simulink model "sampleModel1769"  (R2023a)
settings: Solver=VariableStepAuto  StartTime=0.0  StopTime=10.0  RelTol=1e-3
libraries: hdlsllib x5, simulink x1
settings Model: Creator=user1  LastModifiedBy=user1

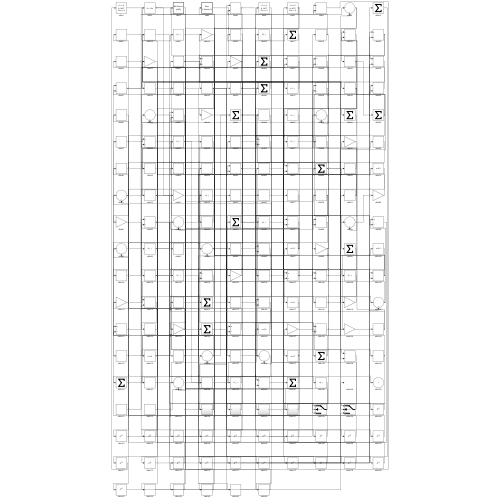
[thumbnail: Simulink's stored preview of the top-level diagram]
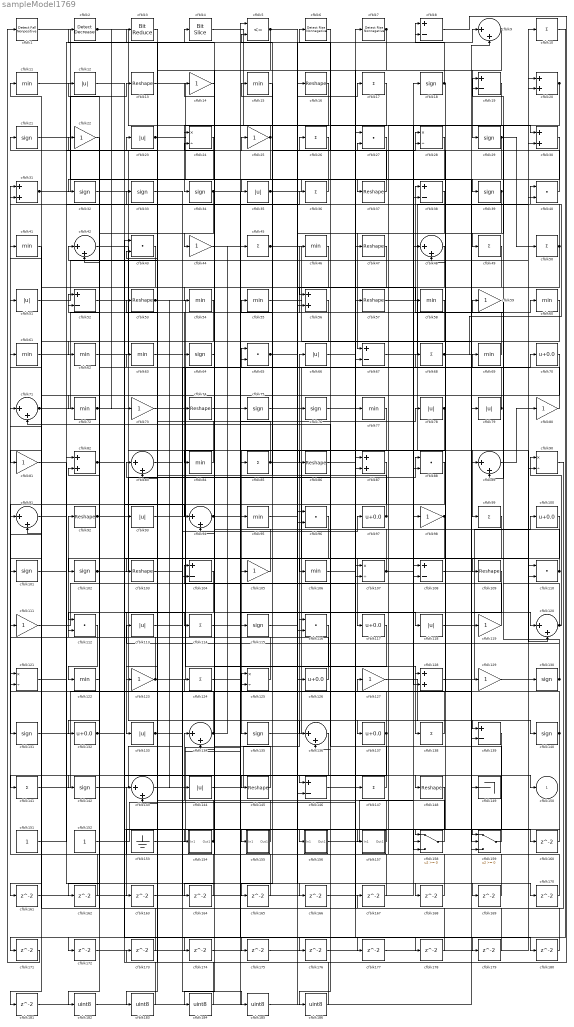
== system sampleModel1769 ==
  cfblk1 : hdlsllib/Logic and Bit Operations/Detect Fall Nonpositive  vinit=0  OutDataTypeStr=boolean
  cfblk{10,17,26,36,45,49..50,68,85,99,114,124,138,141,147} (15 alike) : Sum  Inputs=+
  cfblk{70,97,100,117,126,132,137} (7 alike) : Bias  Bias=0.0  SaturateOnIntegerOverflow=off
  cfblk{18,21,29,32..34,39,64,75..76,101..102,115,130..131,135,140,142} (18 alike) : Signum
  cfblk{13,16,37,47,53,57,74,86,92,103,109,145,148} (13 alike) : Reshape
  cfblk{8,19,38,52,67,104,108,139,146} (9 alike) : Sum  Inputs=+-
  cfblk{14,22,25,44,59,73,80..81,98,105,111,119,123,127,129} (15 alike) : Gain
  cfblk{11,15,41,46,54..55,58,60..63,69,72,77,84,95,106,122} (18 alike) : MinMax
  cfblk{24,28,90,107,121,125} (6 alike) : Product  Inputs=*/  RndMeth=Zero  SaturateOnIntegerOverflow=on
  cfblk{27,40,43,65,88,96,110,112,116} (9 alike) : DotProduct  OutDataTypeStr=Inherit: Inherit via internal rule
  cfblk{12,23,35,51,66,78..79,93,113,118,133,144} (12 alike) : Abs  SaturateOnIntegerOverflow=off
  cfblk{9,42,48,71,83,89,91,94,120,134,136,143} (12 alike) : Sum  Inputs=|++
  cfblk{20,30..31,56,82,87,128} (7 alike) : Sum
  cfblk149 : Terminator
  cfblk151 : Constant  SampleTime=-1
  cfblk152 : Constant  SampleTime=-1
  cfblk153 : Ground
  cfblk154 : Subsystem
      settings: LibrarySourceBlock=|
      | hdlsllib/Ports &
      | Subsystems/Subsystem
  cfblk155 : Subsystem
      settings: LibrarySourceBlock=|
      | hdlsllib/Ports &
      | Subsystems/Subsystem
  cfblk156 : Subsystem
      settings: LibrarySourceBlock=|
      | hdlsllib/Ports &
      | Subsystems/Subsystem
  cfblk157 : Subsystem
      settings: LibrarySourceBlock=|
      | hdlsllib/Ports &
      | Subsystems/Subsystem
  cfblk158 : Switch  SaturateOnIntegerOverflow=off  InputSameDT=off
  cfblk159 : Switch  SaturateOnIntegerOverflow=off  InputSameDT=off
  cfblk{160..181} (22 alike) : Delay  SampleTime=1
  cfblk{182..186} (5 alike) : DataTypeConversion  OutDataTypeStr=uint8  SaturateOnIntegerOverflow=off  RndMeth=Floor
  cfblk2 : simulink/Logic and Bit Operations/Detect Decrease  vinit=0.0  OutDataTypeStr=boolean
      settings: LibrarySourceBlock=|
      | hdlsllib/Logic and Bit
      | Operations/Detect
      | Decrease
  cfblk3 : hdlsllib/Logic and Bit Operations/Bit Reduce  mode=AND
  cfblk4 : hdlsllib/Logic and Bit Operations/Bit Slice  lidx=7  ridx=0
  cfblk5 : RelationalOperator  Operator=<=  OutDataTypeStr=boolean  InputSameDT=off
  cfblk6 : hdlsllib/Logic and Bit Operations/Detect Rise Nonnegative  vinit=0  OutDataTypeStr=boolean
  cfblk7 : hdlsllib/Logic and Bit Operations/Detect Rise Nonnegative  vinit=0  OutDataTypeStr=boolean
  cfblk150 : Outport  VectorParamsAs1DForOutWhenUnconnected=off
  wires:
  cfblk123/1 -> cfblk69/1, cfblk61/1
  cfblk128/1 -> cfblk100/1
  cfblk93/1 -> cfblk60/1
  cfblk77/1 -> cfblk135/1
  cfblk68/1 -> cfblk40/1, cfblk110/2
  cfblk69/1 -> cfblk38/1
  cfblk2/1 -> cfblk30/1, cfblk73/1
  cfblk16/1 -> cfblk34/1
  cfblk157/1(Out1) -> cfblk134/1
  cfblk140/1 -> cfblk68/1, cfblk163/1
  cfblk89/1 -> cfblk80/1
  cfblk85/1 -> cfblk109/1, cfblk8/1, cfblk64/1
  cfblk112/1 -> cfblk122/1
  cfblk97/1 -> cfblk42/1, cfblk21/1, cfblk55/1
  cfblk144/1 -> cfblk66/1
  cfblk31/1 -> cfblk13/1, cfblk28/2
  cfblk26/1 -> cfblk35/1
  cfblk51/1 -> cfblk30/2
  cfblk148/1 -> cfblk31/1
  cfblk133/1 -> cfblk70/1, cfblk83/2
  cfblk38/1 -> cfblk67/1
  cfblk56/1 -> cfblk155/1(In1)
  cfblk88/1 -> cfblk131/1
  cfblk36/1 -> cfblk32/1
  cfblk131/1 -> cfblk79/1
  cfblk34/1 -> cfblk150/1, cfblk72/1, cfblk156/1(In1), cfblk128/1
  cfblk1/1 -> cfblk119/1
  cfblk75/1 -> cfblk16/1
  cfblk32/1 -> cfblk25/1
  cfblk29/1 -> cfblk115/1, cfblk50/1
  cfblk52/1 -> cfblk140/1
  cfblk135/1 -> cfblk10/1
  cfblk145/1 -> cfblk124/1
  cfblk125/1 -> cfblk92/1
  cfblk33/1 -> cfblk136/1
  cfblk136/1 -> cfblk141/1
  cfblk120/1 -> cfblk90/1, cfblk19/1
  cfblk53/1 -> cfblk106/1, cfblk144/1
  cfblk42/1 -> cfblk137/1
  cfblk98/1 -> cfblk117/1, cfblk28/1
  cfblk104/1 -> cfblk133/1
  cfblk23/1 -> cfblk147/1, cfblk77/1
  cfblk127/1 -> cfblk139/1
  cfblk62/1 -> cfblk26/1
  cfblk137/1 -> cfblk127/1, cfblk165/1
  cfblk147/1 -> cfblk83/1
  cfblk11/1 -> cfblk129/1
  cfblk21/1 -> cfblk37/1
  cfblk4/1 -> cfblk98/1
  cfblk45/1 -> cfblk139/2, cfblk58/1
  cfblk102/1 -> cfblk88/1, cfblk175/1
  cfblk153/1 -> cfblk75/1
  cfblk30/1 -> cfblk95/1
  cfblk152/1 -> cfblk7/1
  cfblk142/1 -> cfblk97/1
  cfblk138/1 -> cfblk51/1
  cfblk92/1 -> cfblk93/1, cfblk94/1
  cfblk114/1 -> cfblk118/1
  cfblk155/1(Out1) -> cfblk53/1
  cfblk100/1 -> cfblk102/1
  cfblk5/1 -> cfblk94/2, cfblk168/1
  cfblk65/1 -> cfblk90/2, cfblk5/2
  cfblk154/1(Out1) -> cfblk121/1, cfblk111/1
  cfblk15/1 -> cfblk145/1
  cfblk67/1 -> cfblk20/2
  cfblk79/1 -> cfblk23/1, cfblk22/1
  cfblk141/1 -> cfblk116/1
  cfblk80/1 -> cfblk12/1
  cfblk109/1 -> cfblk142/1
  cfblk132/1 -> cfblk125/1, cfblk158/2
  cfblk129/1 -> cfblk130/1
  cfblk95/1 -> cfblk17/1
  cfblk25/1 -> cfblk54/1, cfblk112/1, cfblk24/1
  cfblk57/1 -> cfblk99/1
  cfblk151/1 -> cfblk82/1
  cfblk27/1 -> cfblk123/1
  cfblk73/1 -> cfblk138/1
  cfblk84/1 -> cfblk33/1
  cfblk72/1 -> cfblk132/1, cfblk120/2, cfblk148/1
  cfblk110/1 -> cfblk74/1, cfblk14/1
  cfblk9/1 -> cfblk84/1, cfblk29/1
  cfblk156/1(Out1) -> cfblk48/1
  cfblk78/1 -> cfblk96/2, cfblk128/2
  cfblk83/1 -> cfblk65/1
  cfblk3/1 -> cfblk103/1
  cfblk12/1 -> cfblk146/1
  cfblk116/1 -> cfblk146/2
  cfblk134/1 -> cfblk82/2, cfblk45/1
  cfblk35/1 -> cfblk39/1, cfblk158/3
  cfblk17/1 -> cfblk136/2
  cfblk76/1 -> cfblk47/1
  cfblk115/1 -> cfblk76/1
  cfblk7/1 -> cfblk87/2, cfblk183/1
  cfblk119/1 -> cfblk104/1
  cfblk159/1 -> cfblk71/2
  cfblk50/1 -> cfblk154/1(In1), cfblk11/1, cfblk19/2
  cfblk96/1 -> cfblk143/2
  cfblk20/1 -> cfblk157/1(In1), cfblk49/1
  cfblk86/1 -> cfblk107/1
  cfblk41/1 -> cfblk81/1
  cfblk28/1 -> cfblk105/1
  cfblk122/1 -> cfblk52/1
  cfblk111/1 -> cfblk57/1
  cfblk130/1 -> cfblk59/1, cfblk113/1
  cfblk61/1 -> cfblk38/2
  cfblk94/1 -> cfblk169/1, cfblk170/1
  cfblk143/1 -> cfblk85/1
  cfblk71/1 -> cfblk46/1, cfblk31/2
  cfblk158/1 -> cfblk4/1
  cfblk55/1 -> cfblk88/2
  cfblk19/1 -> cfblk48/2
  cfblk118/1 -> cfblk120/1
  cfblk106/1 -> cfblk87/1
  cfblk126/1 -> cfblk41/1
  cfblk107/1 -> cfblk18/1, cfblk24/2
  cfblk24/1 -> cfblk42/2
  cfblk13/1 -> cfblk89/1
  cfblk82/1 -> cfblk108/2, cfblk114/1
  cfblk14/1 -> cfblk44/1
  cfblk48/1 -> cfblk86/1
  cfblk99/1 -> cfblk116/2
  cfblk121/1 -> cfblk36/1
  cfblk18/1 -> cfblk158/1, cfblk8/2
  cfblk40/1 -> cfblk15/1
  cfblk49/1 -> cfblk65/2
  cfblk105/1 -> cfblk2/1
  cfblk101/1 -> cfblk9/1
  cfblk37/1 -> cfblk6/1
  cfblk46/1 -> cfblk56/1
  cfblk70/1 -> cfblk91/2
  cfblk124/1 -> cfblk78/1
  cfblk58/1 -> cfblk62/1
  cfblk59/1 -> cfblk89/2
  cfblk108/1 -> cfblk159/2
  cfblk87/1 -> cfblk101/1
  cfblk91/1 -> cfblk27/2
  cfblk39/1 -> cfblk107/2, cfblk56/2
  cfblk146/1 -> cfblk160/1
  cfblk160/1 -> cfblk159/1
  cfblk47/1 -> cfblk161/1
  cfblk161/1 -> cfblk104/2
  cfblk54/1 -> cfblk162/1
  cfblk162/1 -> cfblk91/1
  cfblk163/1 -> cfblk108/1
  cfblk139/1 -> cfblk164/1
  cfblk164/1 -> cfblk143/1
  cfblk165/1 -> cfblk112/2
  cfblk81/1 -> cfblk166/1
  cfblk166/1 -> cfblk67/2
  cfblk90/1 -> cfblk167/1
  cfblk167/1 -> cfblk96/1
  cfblk168/1 -> cfblk134/2
  cfblk169/1 -> cfblk121/2
  cfblk170/1 -> cfblk5/1
  cfblk10/1 -> cfblk171/1
  cfblk171/1 -> cfblk1/1
  cfblk22/1 -> cfblk172/1
  cfblk172/1 -> cfblk40/2
  cfblk8/1 -> cfblk173/1
  cfblk173/1 -> cfblk52/2
  cfblk64/1 -> cfblk174/1
  cfblk174/1 -> cfblk159/3
  cfblk175/1 -> cfblk9/2
  cfblk74/1 -> cfblk176/1
  cfblk176/1 -> cfblk20/1
  cfblk44/1 -> cfblk177/1
  cfblk177/1 -> cfblk110/1
  cfblk113/1 -> cfblk178/1
  cfblk178/1 -> cfblk71/1
  cfblk66/1 -> cfblk179/1
  cfblk179/1 -> cfblk27/1
  cfblk103/1 -> cfblk180/1
  cfblk180/1 -> cfblk3/1
  cfblk60/1 -> cfblk181/1
  cfblk181/1 -> cfblk125/2
  cfblk43/1 -> cfblk182/1
  cfblk182/1 -> cfblk149/1
  cfblk183/1 -> cfblk43/1
  cfblk117/1 -> cfblk184/1
  cfblk184/1 -> cfblk43/2
  cfblk63/1 -> cfblk185/1
  cfblk185/1 -> cfblk126/1
  cfblk6/1 -> cfblk186/1
  cfblk186/1 -> cfblk63/1

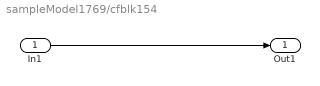
== system sampleModel1769/cfblk154 ==
  In1 : Inport
  Out1 : Outport
  wires:
  In1/1 -> Out1/1

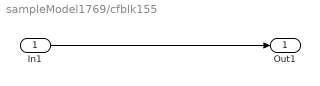
== system sampleModel1769/cfblk155 ==
  In1 : Inport
  Out1 : Outport
  wires:
  In1/1 -> Out1/1

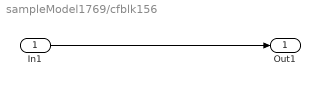
== system sampleModel1769/cfblk156 ==
  In1 : Inport
  Out1 : Outport
  wires:
  In1/1 -> Out1/1

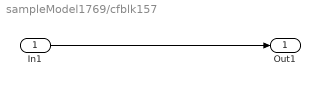
== system sampleModel1769/cfblk157 ==
  In1 : Inport
  Out1 : Outport
  wires:
  In1/1 -> Out1/1
